simulink model "visualize_variables"  (Simulink 9.2)
settings: Solver=FixedStepAuto  StartTime=0.0  StopTime=inf  FixedStep=0.1  RelTol=1e-3
libraries: genomix x3
settings Model: Creator=mtognon  LastModifiedBy=gcorsini
settings DataIOCC: LimitDataPoints=off  SaveFormat=Dataset  SignalLoggingSaveFormat=Dataset
settings OptimizationCC: LifeSpan=auto
settings DebuggingCC: UnderspecifiedInitializationDetection=Simplified  MergeDetectMultiDrivingBlocksExec=error  FcnCallInpInsideContextMsg=error  StateNameClashWarn=none  SFUnexpectedBacktrackingDiag=error  SFNoUnconditionalDefaultTransitionDiag=error  SFExecutionAtInitializationDiag=warning
settings HardwareCC: ProdBitPerPointer=64  ProdBitPerSizeT=64  ProdBitPerPtrDiffT=64  ProdLargestAtomicFloat=Float  ProdIntDivRoundTo=Zero  ProdEndianess=LittleEndian  ProdWordSize=64  ProdHWDeviceType=Intel->x86-64 (Windows64)
settings ModelReferenceCC: PropagateSignalLabelsOutOfModel=on
settings CodeAppCC: StateflowObjectComments=off
settings GRTTargetCC: TargetLangStandard=C99 (ISO)  GeneratePreprocessorConditionals=Use local settings  CombineOutputUpdateFcns=on  GRTInterface=off
settings ConfigComp: CovMetricSettings=dwe  CovHtmlReporting=off  CovSaveCumulativeToWorkspaceVar=off  CovSaveSingleToWorkspaceVar=off  CovExternalEMLEnable=on

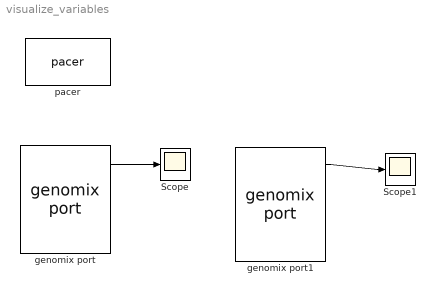
== system visualize_variables ==
  Scope : Scope
  Scope1 : Scope
  genomix port : genomix/genomix port  host=localhost  component=pom  port=frame  subport=robot  sigtype=value  timetype=periodic  period=0.1  siglist="[{\"name\":\"frame.pos\",\"type\":\"value\",\"size\":3}]"
      settings: AttributesFormatString=pom/frame  SourceProductName=genomix
  genomix port1 : genomix/genomix port  host=localhost  component=rotorcraft  port=rotor_measure  sigtype=value  timetype=periodic  period=0.1  siglist="[{\"name\":\"rotor_measure\",\"type\":\"value\",\"size\":80}]"
      settings: AttributesFormatString=rotorcraft/rotor_measure  SourceProductName=genomix
  pacer : genomix/pacer  Priority=0  catchup=off
      settings: SourceProductName=genomix
  wires:
  genomix port/1 -> Scope/1
  genomix port1/1 -> Scope1/1
